simulink model "two_DOF_planar_arm"  (R2020b)
settings: Solver=VariableStepAuto  StartTime=0.0  StopTime=100  RelTol=1e-3
settings Model: Creator=hp  LastModifiedBy=hp
settings DataIOCC: ReturnWorkspaceOutputs=off
settings DebuggingCC: ArithmeticOperatorsInVariantConditions=warning
settings SFSimCC: SimUseLocalCustomCode=off  CustomCodeUndefinedFunction=UseInterfaceOnly
settings RTWCC: RTWUseLocalCustomCode=off

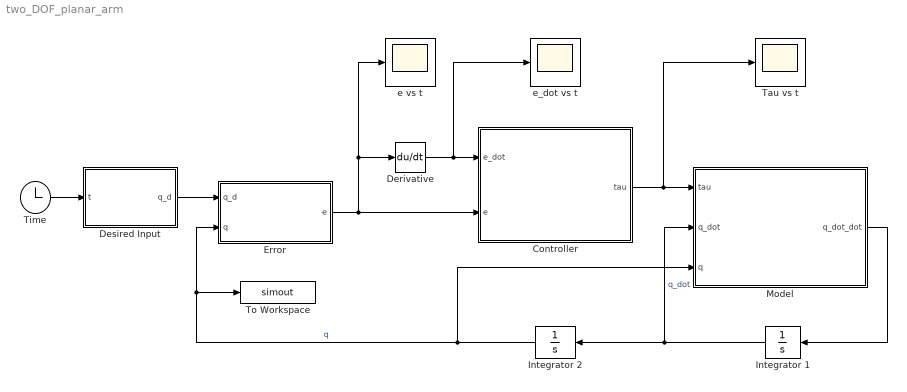
== system two_DOF_planar_arm ==
  Controller : MATLAB Function  TreatAsAtomicUnit=on
  Derivative : Derivative
  Desired Input : MATLAB Function  TreatAsAtomicUnit=on
  Error : MATLAB Function  TreatAsAtomicUnit=on
  Integrator 1 : Integrator  InitialCondition=[0;0]
  Integrator 2 : Integrator  InitialCondition=[0;0]
  Model : MATLAB Function  TreatAsAtomicUnit=on
  Tau vs t : Scope
  Time : Clock
  To Workspace : ToWorkspace  VariableName=simout  SampleTime=-1
      settings: Save2DSignal=2-D array (concatenate along first dimension)
  e vs t : Scope
  e_dot vs t : Scope
  wires:
  Time/1 -> Desired Input/1(t)
  Desired Input/1(q_d) -> Error/1(q_d)
  Error/1(e) -> Controller/2(e), Derivative/1, e vs t/1
  Derivative/1 -> e_dot vs t/1, Controller/1(e_dot)
  Controller/1(tau) -> Tau vs t/1, Model/1(tau)
  Model/1(q_dot_dot) -> Integrator 1/1
  Integrator 1/1 -> Model/2(q_dot), Integrator 2/1  "q_dot"
  Integrator 2/1 -> Model/3(q), Error/2(q), To Workspace/1  "q"

== matlab function two_DOF_planar_arm/Error ==
  data: q_d input; q input; e output
function e = fcn(q_d,q)

e = q - q_d;

end

== matlab function two_DOF_planar_arm/Desired Input ==
  data: t input; q_d output
function q_d = fnc(t)
%% Case A
   
q_d = [pi/3;pi/4];

%% Case B
   
%q_d = [sin(t);cos(t)];

end

== matlab function two_DOF_planar_arm/Controller ==
  data: e_dot input; e input; tau output
function tau = fcn(e_dot,e)

k1=1;
k2=1;
tau = -(k1*e)-(k2*e_dot);

end

== matlab function two_DOF_planar_arm/Model ==
  data: tau input; q_dot_dot output; q_dot input; q input
function q_dot_dot  = fcn(tau,q_dot,q)

m1=1; m2=1; l1=1; l2=1; g=9.8;
theta1_dot=q_dot(1,1); theta2_dot=q_dot(2,1);
theta1=q(1,1); theta2=q(2,1);

mass_matrix = [ ((m1+m2)*l1*l1)+(m2*l2*l2)+(2*m2*l1*l2*cos(theta2)) , (m2*l2*l2)+(m2*l1*l2*cos(theta2)) ;
                (m2*l2*l2)+(m2*l1*l2*cos(theta2))                   , (m2*l2*l2)                       ];
             
coriolis_term = [ -m2*l1*l2*((2*theta1_dot*theta2_dot)+(theta2_dot*theta2_dot))*sin(theta2) ;
                               m2*l1*l2*theta1_dot*theta1_dot*sin(theta2)                  ];
           
gravity_term = [ ((m1+m2)*g*l1*cos(theta1))+(m2*g*l2*cos(theta1+theta2)) ;
                  m2*g*l2*cos(theta1+theta2)                            ];
              
q_dot_dot = mass_matrix \ (tau-coriolis_term-gravity_term);           
                                                                                        
end
